simulink model "project2"  (R2019a)
settings: Solver=VariableStepAuto  StartTime=0.0  StopTime=10.0  RelTol=1e-3
values from neighbouring files (symbols this model uses):
  x = input(prompt)    [project2_script.m]
settings Model: Creator=YosifUonis  LastModifiedBy=YosifUonis

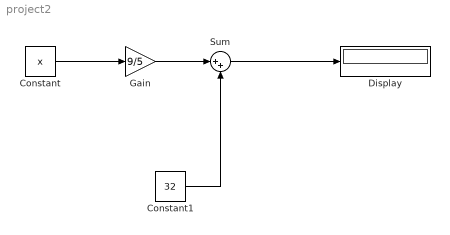
== system project2 ==
  Constant : Constant  Value=x
  Constant1 : Constant  Value=32
  Display : Display
  Gain : Gain  Gain=9/5
  Sum : Sum  Inputs=|++
  wires:
  Constant/1 -> Gain/1
  Constant1/1 -> Sum/2
  Gain/1 -> Sum/1
  Sum/1 -> Display/1
